simulink model "cruise_control_harness"  (Simulink 7.8)
settings: Solver=FixedStepDiscrete  SolverMode=SingleTasking  StartTime=0.0  StopTime=50  FixedStep=0.01  RelTol=1e-3  AbsTol=1e-6
model workspace (MAT data in the model file):
  converter_data = [0  137.465208994  2.232; 0.1  137.065019157  2.075; 0.2  135.864449646  1.975; 0.3  135.664354728  1.846; 0.4  137.565256453  1.72; 0.5  140.366585312  1.564; 0.6  145.268910814  1.409; 0.7  152.872517717  1.254; 0.8  162.9773111  1.096; 0.81  164.27792807  1.08; 0.82  166.178829795  1.061; 0.83  167.979684062  1.043; 0.84  170.080680706  1.028; 0.85  172.781962105  1.012; 0.86  175.383196045  1.002; 0.87  179.585189333  1.002; 0.88  183.587087703  1.001; 0.89  189.890077635  0.998; 0.9  197.693779455  0.999; 0.92  215.902417037  1.001; 0.94  244.515990379  1.002]
  emap = [-40  -44  -49  -53  -57  -61  -65  -70  -74  -78  -82; 215  117  85  66  44  29  10  -2  -13  -22  -32; 245  208  178  148  122  104  85  66  48  33  18; 264  260  241  219  193  167  152  133  119  96  85; 264  279  282  275  260  238  223  208  189  171  152; 267  290  293  297  290  275  260  256  234  212  193; 267  297  305  305  305  301  293  282  267  249  226; 267  301  308  312  319  323  319  316  297  279  253; 267  301  312  319  327  327  327  327  312  293  267; 267  301  312  319  327  334  334  334  319  305  275]
  Iei = 0.0219914882836
  nevec = [800 1200 1600 2000 2400 2800 3200 3600 4000 4400 4800]
  p0 = 0.07934
  p1 = 0.07934
  thvec = [0; 20; 30; 40; 50; 60; 70; 80; 90; 100]
  vehicledata : num (value not decoded)
values from neighbouring files (symbols this model uses):
  cruise_ki = 0.01    [cruise_control_data.m]    (also in fxpdata_simulinkpackage.mat)
  cruise_kp = 0.02    [cruise_control_data.m]    (also in fxpdata_simulinkpackage.mat)
  target_max = 100    [cruise_control_data.m]    (also in fxpdata_simulinkpackage.mat)
  target_min = 30    [cruise_control_data.m]    (also in fxpdata_simulinkpackage.mat)
  throt_max = 100    [cruise_control_data.m]    (also in fxpdata_simulinkpackage.mat)
  throt_min = 0    [cruise_control_data.m]    (also in fxpdata_simulinkpackage.mat)
  vel_dec = 1    [cruise_control_data.m]    (also in fxpdata_simulinkpackage.mat)
  vel_inc = 1    [cruise_control_data.m]    (also in fxpdata_simulinkpackage.mat)
undefined symbols (not defined in the file or in its folder): DiscIntNeverNeededParam, sigbuilder_block
libraries: simulink x2
settings Model: MinMaxOverflowLogging=MinMaxAndOverflow  SldvGeneratedHarnessModel=TestUnitModel=cruise_control|  Creator=The MathWorks Inc.  LastModifiedBy=itoy  RecordCoverage=on  CovSaveName=covdata_cc  CovMetricSettings=dcmtroe  CovHTMLOptions=-aTS=1 -bRG=1 -bTC=0 -hTR=0 -nFC=0 -scm=1 -bcm=1  CovModelRefEnable=off  CovExternalEMLEnable=on  ExtModeTrigMode=oneshot  ExtModeArmWhenConnect=off  ExtModeAutoUpdateStatusClock=off
settings DataIOCC: LimitDataPoints=off  SaveFormat=StructureWithTime  SaveOutput=off  SignalLogging=off  DSMLogging=off  SaveTime=off  SignalLoggingName=mysig
settings OptimizationCC: InlineParams=on  UseIntDivNetSlope=on  InlineInvariantSignals=on  EnhancedBackFolding=on  EfficientFloat2IntCast=on  OptimizeModelRefInitCode=on  LifeSpan=1
settings DebuggingCC: SignalInfNanChecking=error  SaveWithParameterizedLinksMsg=none  CheckExecutionContextPreStartOutputMsg=on  CheckExecutionContextRuntimeOutputMsg=on  SolverPrmCheckMsg=none  InheritedTsInSrcMsg=none  SingleTaskRateTransMsg=error  IntegerOverflowMsg=error  UniqueDataStoreMsg=error  BusObjectLabelMismatch=error  RootOutportRequireBusObject=error  AssertControl=DisableAll  StrictBusMsg=ErrorOnBusTreatedAsVector  BusNameAdapt=ErrorWithoutRepair  NonBusSignalsTreatedAsBus=error  LoggingUnavailableSignals=none
settings HardwareCC: ProdIntDivRoundTo=Zero  ProdEndianess=LittleEndian  ProdHWDeviceType=NEC->V850  TargetIntDivRoundTo=Zero  TargetEndianess=LittleEndian  TargetHWDeviceType=MATLAB Host
settings ModelReferenceCC: ModelReferenceNumInstancesAllowed=Single
settings SFSimCC: SFSimEcho=off  SimParseCustomCode=off
settings RTWCC: SystemTargetFile=ert.tlc  TemplateMakefile=ert_default_tmf  Description=Real-Time Workshop Embedded Coder  GenerateReport=on  ProcessScript=ert_make_rtw_hook  IncludeHyperlinkInReport=on  LaunchReport=on  IncludeERTFirstTime=on  RTWCompilerOptimization=On
settings CodeAppCC: IgnoreCustomStorageClasses=off
settings ERTTargetCC: MultiwordLength=2048  GenerateSampleERTMain=on  GenerateErtSFunction=on  CreateSILPILBlock=SIL  InlinedParameterPlacement=NonHierarchical  ERTCustomFileTemplate=example_file_process.tlc  ConvertIfToSwitch=off  SuppressUnreachableDefaultCases=off
settings ConfigComp: Description=Design Verifier Custom Configuration Component  DVMaxProcessTime=3000  DVDisplayUnsatisfiableObjectives=on  DVModelCoverageObjectives=MCDC  DVMaxTestCaseSteps=500  DVTestSuiteOptimization=CombinedObjectives  DVSaveReport=on

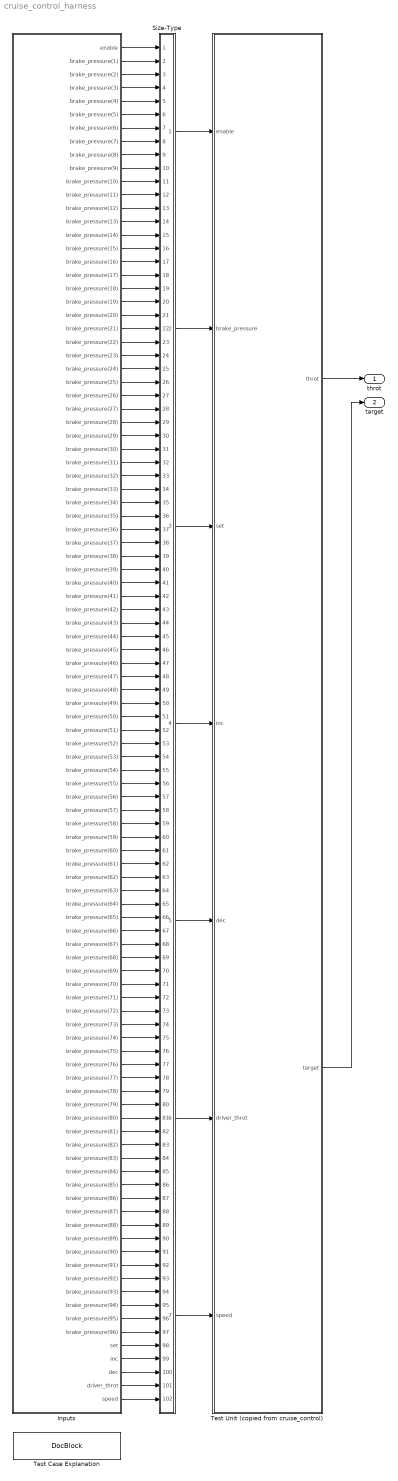
== system cruise_control_harness ==
  Inputs : Subsystem  Tag=STV Subsys  LoadFcn=sigbuilder_block('load',[49.5 50.25 519.75 399.75 ]);  StartFcn=sigbuilder_block('start');  StopFcn=sigbuilder_block('stop');  ClipboardFcn=sigbuilder_block('clipboard');  mask(Sigbuilder block){}
      mask init:
      | if ~strcmp(get_param(bdroot(gcb),'SimulationStatus'),'stopped'),tuvar = sigbuilder_block('maskInit'); end
      settings: CopyFcn=sigbuilder_block('copy');  DeleteFcn=sigbuilder_block('delete');  ModelCloseFcn=sigbuilder_block('modelClose');  PreSaveFcn=sigbuilder_block('preSave');  NameChangeFcn=sigbuilder_block('namechange');  OpenFcn=sigbuilder_block('open');  CloseFcn=sigbuilder_block('close');
      mask Display: plot(0, 0, 100, 100,[2, 2, 32, 32, 2], [68, 8, 8, 68, 68],[32, 2], [38, 38], [32, 19, 2],[53, 60, 44], [32, 17, 17, 2],[16, 16, 31, 31]);txt = getActiveGroup(gcbh);text(2, 100, txt,'verticalAlignment', 'top');
  Size-Type : Subsystem
  Test Case Explanation : simulink/Model-Wide Utilities/DocBlock  DocumentType=Text
  Test Unit (copied from cruise_control) : Subsystem
  throt : Outport  PortDimensions=[1 1]
  target : Outport  Port=2  PortDimensions=[1 1]
  wires:
  Inputs/1(enable) -> Size-Type/1(In1)
  Size-Type/1(Out1) -> Test Unit (copied from cruise_control)/1(enable)
  Inputs/2(brake_pressure(1)) -> Size-Type/2(In2)
  Inputs/3(brake_pressure(2)) -> Size-Type/3(In3)
  Inputs/4(brake_pressure(3)) -> Size-Type/4(In4)
  Inputs/5(brake_pressure(4)) -> Size-Type/5(In5)
  Inputs/6(brake_pressure(5)) -> Size-Type/6(In6)
  Inputs/7(brake_pressure(6)) -> Size-Type/7(In7)
  Inputs/8(brake_pressure(7)) -> Size-Type/8(In8)
  Inputs/9(brake_pressure(8)) -> Size-Type/9(In9)
  Inputs/10(brake_pressure(9)) -> Size-Type/10(In10)
  Inputs/11(brake_pressure(10)) -> Size-Type/11(In11)
  Inputs/12(brake_pressure(11)) -> Size-Type/12(In12)
  Inputs/13(brake_pressure(12)) -> Size-Type/13(In13)
  Inputs/14(brake_pressure(13)) -> Size-Type/14(In14)
  Inputs/15(brake_pressure(14)) -> Size-Type/15(In15)
  Inputs/16(brake_pressure(15)) -> Size-Type/16(In16)
  Inputs/17(brake_pressure(16)) -> Size-Type/17(In17)
  Inputs/18(brake_pressure(17)) -> Size-Type/18(In18)
  Inputs/19(brake_pressure(18)) -> Size-Type/19(In19)
  Inputs/20(brake_pressure(19)) -> Size-Type/20(In20)
  Inputs/21(brake_pressure(20)) -> Size-Type/21(In21)
  Inputs/22(brake_pressure(21)) -> Size-Type/22(In22)
  Inputs/23(brake_pressure(22)) -> Size-Type/23(In23)
  Inputs/24(brake_pressure(23)) -> Size-Type/24(In24)
  Inputs/25(brake_pressure(24)) -> Size-Type/25(In25)
  Inputs/26(brake_pressure(25)) -> Size-Type/26(In26)
  Inputs/27(brake_pressure(26)) -> Size-Type/27(In27)
  Inputs/28(brake_pressure(27)) -> Size-Type/28(In28)
  Inputs/29(brake_pressure(28)) -> Size-Type/29(In29)
  Inputs/30(brake_pressure(29)) -> Size-Type/30(In30)
  Inputs/31(brake_pressure(30)) -> Size-Type/31(In31)
  Inputs/32(brake_pressure(31)) -> Size-Type/32(In32)
  Inputs/33(brake_pressure(32)) -> Size-Type/33(In33)
  Inputs/34(brake_pressure(33)) -> Size-Type/34(In34)
  Inputs/35(brake_pressure(34)) -> Size-Type/35(In35)
  Inputs/36(brake_pressure(35)) -> Size-Type/36(In36)
  Inputs/37(brake_pressure(36)) -> Size-Type/37(In37)
  Inputs/38(brake_pressure(37)) -> Size-Type/38(In38)
  Inputs/39(brake_pressure(38)) -> Size-Type/39(In39)
  Inputs/40(brake_pressure(39)) -> Size-Type/40(In40)
  Inputs/41(brake_pressure(40)) -> Size-Type/41(In41)
  Inputs/42(brake_pressure(41)) -> Size-Type/42(In42)
  Inputs/43(brake_pressure(42)) -> Size-Type/43(In43)
  Inputs/44(brake_pressure(43)) -> Size-Type/44(In44)
  Inputs/45(brake_pressure(44)) -> Size-Type/45(In45)
  Inputs/46(brake_pressure(45)) -> Size-Type/46(In46)
  Inputs/47(brake_pressure(46)) -> Size-Type/47(In47)
  Inputs/48(brake_pressure(47)) -> Size-Type/48(In48)
  Inputs/49(brake_pressure(48)) -> Size-Type/49(In49)
  Inputs/50(brake_pressure(49)) -> Size-Type/50(In50)
  Inputs/51(brake_pressure(50)) -> Size-Type/51(In51)
  Inputs/52(brake_pressure(51)) -> Size-Type/52(In52)
  Inputs/53(brake_pressure(52)) -> Size-Type/53(In53)
  Inputs/54(brake_pressure(53)) -> Size-Type/54(In54)
  Inputs/55(brake_pressure(54)) -> Size-Type/55(In55)
  Inputs/56(brake_pressure(55)) -> Size-Type/56(In56)
  Inputs/57(brake_pressure(56)) -> Size-Type/57(In57)
  Inputs/58(brake_pressure(57)) -> Size-Type/58(In58)
  Inputs/59(brake_pressure(58)) -> Size-Type/59(In59)
  Inputs/60(brake_pressure(59)) -> Size-Type/60(In60)
  Inputs/61(brake_pressure(60)) -> Size-Type/61(In61)
  Inputs/62(brake_pressure(61)) -> Size-Type/62(In62)
  Inputs/63(brake_pressure(62)) -> Size-Type/63(In63)
  Inputs/64(brake_pressure(63)) -> Size-Type/64(In64)
  Inputs/65(brake_pressure(64)) -> Size-Type/65(In65)
  Inputs/66(brake_pressure(65)) -> Size-Type/66(In66)
  Inputs/67(brake_pressure(66)) -> Size-Type/67(In67)
  Inputs/68(brake_pressure(67)) -> Size-Type/68(In68)
  Inputs/69(brake_pressure(68)) -> Size-Type/69(In69)
  Inputs/70(brake_pressure(69)) -> Size-Type/70(In70)
  Inputs/71(brake_pressure(70)) -> Size-Type/71(In71)
  Inputs/72(brake_pressure(71)) -> Size-Type/72(In72)
  Inputs/73(brake_pressure(72)) -> Size-Type/73(In73)
  Inputs/74(brake_pressure(73)) -> Size-Type/74(In74)
  Inputs/75(brake_pressure(74)) -> Size-Type/75(In75)
  Inputs/76(brake_pressure(75)) -> Size-Type/76(In76)
  Inputs/77(brake_pressure(76)) -> Size-Type/77(In77)
  Inputs/78(brake_pressure(77)) -> Size-Type/78(In78)
  Inputs/79(brake_pressure(78)) -> Size-Type/79(In79)
  Inputs/80(brake_pressure(79)) -> Size-Type/80(In80)
  Inputs/81(brake_pressure(80)) -> Size-Type/81(In81)
  Inputs/82(brake_pressure(81)) -> Size-Type/82(In82)
  Inputs/83(brake_pressure(82)) -> Size-Type/83(In83)
  Inputs/84(brake_pressure(83)) -> Size-Type/84(In84)
  Inputs/85(brake_pressure(84)) -> Size-Type/85(In85)
  Inputs/86(brake_pressure(85)) -> Size-Type/86(In86)
  Inputs/87(brake_pressure(86)) -> Size-Type/87(In87)
  Inputs/88(brake_pressure(87)) -> Size-Type/88(In88)
  Inputs/89(brake_pressure(88)) -> Size-Type/89(In89)
  Inputs/90(brake_pressure(89)) -> Size-Type/90(In90)
  Inputs/91(brake_pressure(90)) -> Size-Type/91(In91)
  Inputs/92(brake_pressure(91)) -> Size-Type/92(In92)
  Inputs/93(brake_pressure(92)) -> Size-Type/93(In93)
  Inputs/94(brake_pressure(93)) -> Size-Type/94(In94)
  Inputs/95(brake_pressure(94)) -> Size-Type/95(In95)
  Inputs/96(brake_pressure(95)) -> Size-Type/96(In96)
  Inputs/97(brake_pressure(96)) -> Size-Type/97(In97)
  Size-Type/2(Out2) -> Test Unit (copied from cruise_control)/2(brake_pressure)
  Inputs/98(set) -> Size-Type/98(In98)
  Size-Type/3(Out3) -> Test Unit (copied from cruise_control)/3(set)
  Inputs/99(inc) -> Size-Type/99(In99)
  Size-Type/4(Out4) -> Test Unit (copied from cruise_control)/4(inc)
  Inputs/100(dec) -> Size-Type/100(In100)
  Size-Type/5(Out5) -> Test Unit (copied from cruise_control)/5(dec)
  Inputs/101(driver_throt) -> Size-Type/101(In101)
  Size-Type/6(Out6) -> Test Unit (copied from cruise_control)/6(driver_throt)
  Inputs/102(speed) -> Size-Type/102(In102)
  Size-Type/7(Out7) -> Test Unit (copied from cruise_control)/7(speed)
  Test Unit (copied from cruise_control)/1(throt) -> throt/1
  Test Unit (copied from cruise_control)/2(target) -> target/1

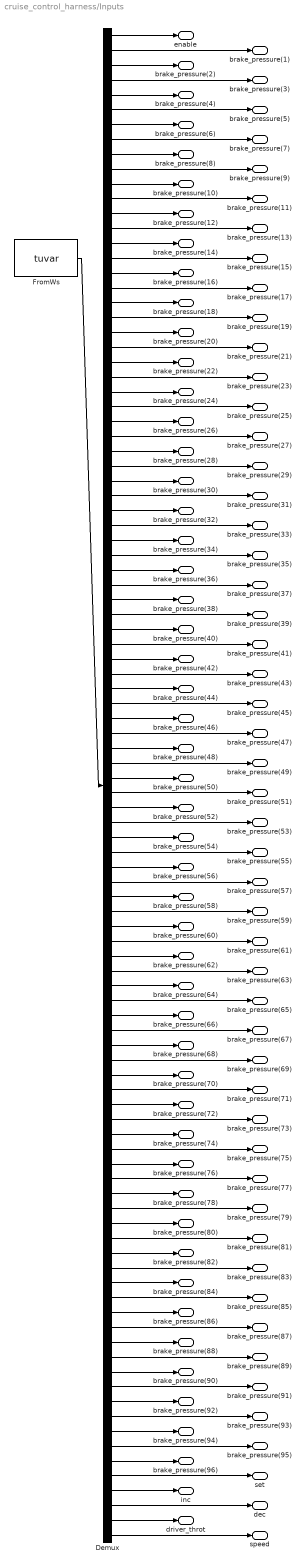
== system cruise_control_harness/Inputs ==
  Demux : Demux  Tag=STV Demux  Outputs=102
  FromWs : FromWorkspace  Tag=STV FromWs  VariableName=tuvar  SampleTime=0  SigBuilderData=DataTag1  VnvData=DataTag2
      SigBuilderData=|
      | dataSet.timeRange = [0 0.01]
      | dataSet.name = 'Test Case 1'
      | sbobj.Name = 'Signal Builder'
      | sbobj.Groups.Name = 'Test Case 1'
      | sbobj.Groups.Signals(1).Name = 'enable'
      | sbobj.Groups.Signals(1).XData = [0 0.01]
      | sbobj.Groups.Signals(1).YData = [0 0]
      | sbobj.Groups.Signals(2).Name = 'brake_pressure(1)'
      | sbobj.Groups.Signals(2).XData = [0 0.01]
      | sbobj.Groups.Signals(2).YData = [0 0]
      | sbobj.Groups.Signals(3).Name = 'brake_pressure(2)'
      | sbobj.Groups.Signals(3).XData = [0 0.01]
      | sbobj.Groups.Signals(3).YData = [0 0]
      | sbobj.Groups.Signals(4).Name = 'brake_pressure(3)'
      | sbobj.Groups.Signals(4).XData = [0 0.01]
      | sbobj.Groups.Signals(4).YData = [0 0]
      | sbobj.Groups.Signals(5).Name = 'brake_pressure(4)'
      | sbobj.Groups.Signals(5).XData = [0 0.01]
      | sbobj.Groups.Signals(5).YData = [0 0]
      | sbobj.Groups.Signals(6).Name = 'brake_pressure(5)'
      | sbobj.Groups.Signals(6).XData = [0 0.01]
      | sbobj.Groups.Signals(6).YData = [0 0]
      | sbobj.Groups.Signals(7).Name = 'brake_pressure(6)'
      | sbobj.Groups.Signals(7).XData = [0 0.01]
      | sbobj.Groups.Signals(7).YData = [0 0]
      | sbobj.Groups.Signals(8).Name = 'brake_pressure(7)'
      | sbobj.Groups.Signals(8).XData = [0 0.01]
      | sbobj.Groups.Signals(8).YData = [0 0]
      | sbobj.Groups.Signals(9).Name = 'brake_pressure(8)'
      | sbobj.Groups.Signals(9).XData = [0 0.01]
      | sbobj.Groups.Signals(9).YData = [0 0]
      | sbobj.Groups.Signals(10).Name = 'brake_pressure(9)'
      | sbobj.Groups.Signals(10).XData = [0 0.01]
      | sbobj.Groups.Signals(10).YData = [0 0]
      | sbobj.Groups.Signals(11).Name = 'brake_pressure(10)'
      | sbobj.Groups.Signals(11).XData = [0 0.01]
      | sbobj.Groups.Signals(11).YData = [0 0]
      | sbobj.Groups.Signals(12).Name = 'brake_pressure(11)'
      | sbobj.Groups.Signals(12).XData = [0 0.01]
      | sbobj.Groups.Signals(12).YData = [0 0]
      | sbobj.Groups.Signals(13).Name = 'brake_pressure(12)'
      | sbobj.Groups.Signals(13).XData = [0 0.01]
      | sbobj.Groups.Signals(13).YData = [0 0]
      | sbobj.Groups.Signals(14).Name = 'brake_pressure(13)'
      | sbobj.Groups.Signals(14).XData = [0 0.01]
      | sbobj.Groups.Signals(14).YData = [0 0]
      | sbobj.Groups.Signals(15).Name = 'brake_pressure(14)'
      | sbobj.Groups.Signals(15).XData = [0 0.01]
      | sbobj.Groups.Signals(15).YData = [0 0]
      | sbobj.Groups.Signals(16).Name = 'brake_pressure(15)'
      | sbobj.Groups.Signals(16).XData = [0 0.01]
      | sbobj.Groups.Signals(16).YData = [0 0]
      | sbobj.Groups.Signals(17).Name = 'brake_pressure(16)'
      | sbobj.Groups.Signals(17).XData = [0 0.01]
      | sbobj.Groups.Signals(17).YData = [0 0]
      | sbobj.Groups.Signals(18).Name = 'brake_pressure(17)'
      | sbobj.Groups.Signals(18).XData = [0 0.01]
      | sbobj.Groups.Signals(18).YData = [0 0]
      | sbobj.Groups.Signals(19).Name = 'brake_pressure(18)'
      | sbobj.Groups.Signals(19).XData = [0 0.01]
      | sbobj.Groups.Signals(19).YData = [0 0]
      | sbobj.Groups.Signals(20).Name = 'brake_pressure(19)'
      | sbobj.Groups.Signals(20).XData = [0 0.01]
      | sbobj.Groups.Signals(20).YData = [0 0]
      | sbobj.Groups.Signals(21).Name = 'brake_pressure(20)'
      | sbobj.Groups.Signals(21).XData = [0 0.01]
      | sbobj.Groups.Signals(21).YData = [0 0]
      | sbobj.Groups.Signals(22).Name = 'brake_pressure(21)'
      | sbobj.Groups.Signals(22).XData = [0 0.01]
      | sbobj.Groups.Signals(22).YData = [0 0]
      | sbobj.Groups.Signals(23).Name = 'brake_pressure(22)'
      | sbobj.Groups.Signals(23).XData = [0 0.01]
      | sbobj.Groups.Signals(23).YData = [0 0]
      | sbobj.Groups.Signals(24).Name = 'brake_pressure(23)'
      | sbobj.Groups.Signals(24).XData = [0 0.01]
      | sbobj.Groups.Signals(24).YData = [0 0]
      | sbobj.Groups.Signals(25).Name = 'brake_pressure(24)'
      | sbobj.Groups.Signals(25).XData = [0 0.01]
      | sbobj.Groups.Signals(25).YData = [0 0]
      | sbobj.Groups.Signals(26).Name = 'brake_pressure(25)'
      | sbobj.Groups.Signals(26).XData = [0 0.01]
      | sbobj.Groups.Signals(26).YData = [0 0]
      | sbobj.Groups.Signals(27).Name = 'brake_pressure(26)'
      | sbobj.Groups.Signals(27).XData = [0 0.01]
      | sbobj.Groups.Signals(27).YData = [0 0]
      | sbobj.Groups.Signals(28).Name = 'brake_pressure(27)'
      | sbobj.Groups.Signals(28).XData = [0 0.01]
      | sbobj.Groups.Signals(28).YData = [0 0]
      | sbobj.Groups.Signals(29).Name = 'brake_pressure(28)'
      | sbobj.Groups.Signals(29).XData = [0 0.01]
      | sbobj.Groups.Signals(29).YData = [0 0]
      | sbobj.Groups.Signals(30).Name = 'brake_pressure(29)'
      | sbobj.Groups.Signals(30).XData = [0 0.01]
      | sbobj.Groups.Signals(30).YData = [0 0]
      | sbobj.Groups.Signals(31).Name = 'brake_pressure(30)'
      | sbobj.Groups.Signals(31).XData = [0 0.01]
      | sbobj.Groups.Signals(31).YData = [0 0]
      | sbobj.Groups.Signals(32).Name = 'brake_pressure(31)'
      | sbobj.Groups.Signals(32).XData = [0 0.01]
      | sbobj.Groups.Signals(32).YData = [0 0]
      | sbobj.Groups.Signals(33).Name = 'brake_pressure(32)'
      | sbobj.Groups.Signals(33).XData = [0 0.01]
      | sbobj.Groups.Signals(33).YData = [0 0]
      | sbobj.Groups.Signals(34).Name = 'brake_pressure(33)'
      | sbobj.Groups.Signals(34).XData = [0 0.01]
      | sbobj.Groups.Signals(34).YData = [0 0]
      | sbobj.Groups.Signals(35).Name = 'brake_pressure(34)'
      | sbobj.Groups.Signals(35).XData = [0 0.01]
      | sbobj.Groups.Signals(35).YData = [0 0]
      | sbobj.Groups.Signals(36).Name = 'brake_pressure(35)'
      | sbobj.Groups.Signals(36).XData = [0 0.01]
      | sbobj.Groups.Signals(36).YData = [0 0]
      | sbobj.Groups.Signals(37).Name = 'brake_pressure(36)'
      | sbobj.Groups.Signals(37).XData = [0 0.01]
      | sbobj.Groups.Signals(37).YData = [0 0]
      | sbobj.Groups.Signals(38).Name = 'brake_pressure(37)'
      | sbobj.Groups.Signals(38).XData = [0 0.01]
      | sbobj.Groups.Signals(38).YData = [0 0]
      | sbobj.Groups.Signals(39).Name = 'brake_pressure(38)'
      | sbobj.Groups.Signals(39).XData = [0 0.01]
      | sbobj.Groups.Signals(39).YData = [0 0]
      | sbobj.Groups.Signals(40).Name = 'brake_pressure(39)'
      | sbobj.Groups.Signals(40).XData = [0 0.01]
      | sbobj.Groups.Signals(40).YData = [0 0]
      | sbobj.Groups.Signals(41).Name = 'brake_pressure(40)'
      | sbobj.Groups.Signals(41).XData = [0 0.01]
      | sbobj.Groups.Signals(41).YData = [0 0]
      | sbobj.Groups.Signals(42).Name = 'brake_pressure(41)'
      | sbobj.Groups.Signals(42).XData = [0 0.01]
      | sbobj.Groups.Signals(42).YData = [0 0]
      | sbobj.Groups.Signals(43).Name = 'brake_pressure(42)'
      | sbobj.Groups.Signals(43).XData = [0 0.01]
      | sbobj.Groups.Signals(43).YData = [0 0]
      | sbobj.Groups.Signals(44).Name = 'brake_pressure(43)'
      | sbobj.Groups.Signals(44).XData = [0 0.01]
      | sbobj.Groups.Signals(44).YData = [0 0]
      | sbobj.Groups.Signals(45).Name = 'brake_pressure(44)'
      | sbobj.Groups.Signals(45).XData = [0 0.01]
      | sbobj.Groups.Signals(45).YData = [0 0]
      | sbobj.Groups.Signals(46).Name = 'brake_pressure(45)'
      | sbobj.Groups.Signals(46).XData = [0 0.01]
      | sbobj.Groups.Signals(46).YData = [0 0]
      | sbobj.Groups.Signals(47).Name = 'brake_pressure(46)'
      | sbobj.Groups.Signals(47).XData = [0 0.01]
      | sbobj.Groups.Signals(47).YData = [0 0]
      | sbobj.Groups.Signals(48).Name = 'brake_pressure(47)'
      | sbobj.Groups.Signals(48).XData = [0 0.01]
      | sbobj.Groups.Signals(48).YData = [0 0]
      | sbobj.Groups.Signals(49).Name = 'brake_pressure(48)'
      | sbobj.Groups.Signals(49).XData = [0 0.01]
      | sbobj.Groups.Signals(49).YData = [0 0]
      | sbobj.Groups.Signals(50).Name = 'brake_pressure(49)'
      | sbobj.Groups.Signals(50).XData = [0 0.01]
      | sbobj.Groups.Signals(50).YData = [0 0]
      | sbobj.Groups.Signals(51).Name = 'brake_pressure(50)'
      | sbobj.Groups.Signals(51).XData = [0 0.01]
      | sbobj.Groups.Signals(51).YData = [0 0]
      | sbobj.Groups.Signals(52).Name = 'brake_pressure(51)'
      | sbobj.Groups.Signals(52).XData = [0 0.01]
      | sbobj.Groups.Signals(52).YData = [0 0]
      | sbobj.Groups.Signals(53).Name = 'brake_pressure(52)'
      | sbobj.Groups.Signals(53).XData = [0 0.01]
      | sbobj.Groups.Signals(53).YData = [0 0]
      | sbobj.Groups.Signals(54).Name = 'brake_pressure(53)'
      | sbobj.Groups.Signals(54).XData = [0 0.01]
      | sbobj.Groups.Signals(54).YData = [0 0]
      | sbobj.Groups.Signals(55).Name = 'brake_pressure(54)'
      | sbobj.Groups.Signals(55).XData = [0 0.01]
      | sbobj.Groups.Signals(55).YData = [0 0]
      | sbobj.Groups.Signals(56).Name = 'brake_pressure(55)'
      | sbobj.Groups.Signals(56).XData = [0 0.01]
      | sbobj.Groups.Signals(56).YData = [0 0]
      | sbobj.Groups.Signals(57).Name = 'brake_pressure(56)'
      | sbobj.Groups.Signals(57).XData = [0 0.01]
      | sbobj.Groups.Signals(57).YData = [0 0]
      | sbobj.Groups.Signals(58).Name = 'brake_pressure(57)'
      | sbobj.Groups.Signals(58).XData = [0 0.01]
      | sbobj.Groups.Signals(58).YData = [0 0]
      | sbobj.Groups.Signals(59).Name = 'brake_pressure(58)'
      | sbobj.Groups.Signals(59).XData = [0 0.01]
      | sbobj.Groups.Signals(59).YData = [0 0]
      | sbobj.Groups.Signals(60).Name = 'brake_pressure(59)'
      | sbobj.Groups.Signals(60).XData = [0 0.01]
      | sbobj.Groups.Signals(60).YData = [0 0]
      | sbobj.Groups.Signals(61).Name = 'brake_pressure(60)'
      | sbobj.Groups.Signals(61).XData = [0 0.01]
      | sbobj.Groups.Signals(61).YData = [0 0]
      | sbobj.Groups.Signals(62).Name = 'brake_pressure(61)'
      | sbobj.Groups.Signals(62).XData = [0 0.01]
      | sbobj.Groups.Signals(62).YData = [0 0]
      | sbobj.Groups.Signals(63).Name = 'brake_pressure(62)'
      | sbobj.Groups.Signals(63).XData = [0 0.01]
      | sbobj.Groups.Signals(63).YData = [0 0]
      | sbobj.Groups.Signals(64).Name = 'brake_pressure(63)'
      | sbobj.Groups.Signals(64).XData = [0 0.01]
      | sbobj.Groups.Signals(64).YData = [0 0]
      | sbobj.Groups.Signals(65).Name = 'brake_pressure(64)'
      | sbobj.Groups.Signals(65).XData = [0 0.01]
      | sbobj.Groups.Signals(65).YData = [0 0]
      | sbobj.Groups.Signals(66).Name = 'brake_pressure(65)'
      | sbobj.Groups.Signals(66).XData = [0 0.01]
      | sbobj.Groups.Signals(66).YData = [0 0]
      | sbobj.Groups.Signals(67).Name = 'brake_pressure(66)'
      | sbobj.Groups.Signals(67).XData = [0 0.01]
      | sbobj.Groups.Signals(67).YData = [0 0]
      | sbobj.Groups.Signals(68).Name = 'brake_pressure(67)'
      | sbobj.Groups.Signals(68).XData = [0 0.01]
      | sbobj.Groups.Signals(68).YData = [0 0]
      | sbobj.Groups.Signals(69).Name = 'brake_pressure(68)'
      | sbobj.Groups.Signals(69).XData = [0 0.01]
      | sbobj.Groups.Signals(69).YData = [0 0]
      | sbobj.Groups.Signals(70).Name = 'brake_pressure(69)'
      | sbobj.Groups.Signals(70).XData = [0 0.01]
      | sbobj.Groups.Signals(70).YData = [0 0]
      | sbobj.Groups.Signals(71).Name = 'brake_pressure(70)'
      | sbobj.Groups.Signals(71).XData = [0 0.01]
      | sbobj.Groups.Signals(71).YData = [0 0]
      | sbobj.Groups.Signals(72).Name = 'brake_pressure(71)'
      | sbobj.Groups.Signals(72).XData = [0 0.01]
      | sbobj.Groups.Signals(72).YData = [0 0]
      | sbobj.Groups.Signals(73).Name = 'brake_pressure(72)'
      | sbobj.Groups.Signals(73).XData = [0 0.01]
      | sbobj.Groups.Signals(73).YData = [0 0]
      | sbobj.Groups.Signals(74).Name = 'brake_pressure(73)'
      | sbobj.Groups.Signals(74).XData = [0 0.01]
      | sbobj.Groups.Signals(74).YData = [0 0]
      | sbobj.Groups.Signals(75).Name = 'brake_pressure(74)'
      | sbobj.Groups.Signals(75).XData = [0 0.01]
      | sbobj.Groups.Signals(75).YData = [0 0]
      | sbobj.Groups.Signals(76).Name = 'brake_pressure(75)'
      | sbobj.Groups.Signals(76).XData = [0 0.01]
      | sbobj.Groups.Signals(76).YData = [0 0]
      | sbobj.Groups.Signals(77).Name = 'brake_pressure(76)'
      | sbobj.Groups.Signals(77).XData = [0 0.01]
      | sbobj.Groups.Signals(77).YData = [0 0]
      | sbobj.Groups.Signals(78).Name = 'brake_pressure(77)'
      | sbobj.Groups.Signals(78).XData = [0 0.01]
      | sbobj.Groups.Signals(78).YData = [0 0]
      | sbobj.Groups.Signals(79).Name = 'brake_pressure(78)'
      | sbobj.Groups.Signals(79).XData = [0 0.01]
      | sbobj.Groups.Signals(79).YData = [0 0]
      | sbobj.Groups.Signals(80).Name = 'brake_pressure(79)'
      | sbobj.Groups.Signals(80).XData = [0 0.01]
      | sbobj.Groups.Signals(80).YData = [0 0]
      | sbobj.Groups.Signals(81).Name = 'brake_pressure(80)'
      | sbobj.Groups.Signals(81).XData = [0 0.01]
      | sbobj.Groups.Signals(81).YData = [0 0]
      | sbobj.Groups.Signals(82).Name = 'brake_pressure(81)'
      | sbobj.Groups.Signals(82).XData = [0 0.01]
      | sbobj.Groups.Signals(82).YData = [0 0]
      | sbobj.Groups.Signals(83).Name = 'brake_pressure(82)'
      | sbobj.Groups.Signals(83).XData = [0 0.01]
      | sbobj.Groups.Signals(83).YData = [0 0]
      | sbobj.Groups.Signals(84).Name = 'brake_pressure(83)'
      | sbobj.Groups.Signals(84).XData = [0 0.01]
      | sbobj.Groups.Signals(84).YData = [0 0]
      | sbobj.Groups.Signals(85).Name = 'brake_pressure(84)'
      | sbobj.Groups.Signals(85).XData = [0 0.01]
      | sbobj.Groups.Signals(85).YData = [0 0]
      | sbobj.Groups.Signals(86).Name = 'brake_pressure(85)'
      | sbobj.Groups.Signals(86).XData = [0 0.01]
      | sbobj.Groups.Signals(86).YData = [0 0]
      | sbobj.Groups.Signals(87).Name = 'brake_pressure(86)'
      | sbobj.Groups.Signals(87).XData = [0 0.01]
      | sbobj.Groups.Signals(87).YData = [0 0]
      | sbobj.Groups.Signals(88).Name = 'brake_pressure(87)'
      | sbobj.Groups.Signals(88).XData = [0 0.01]
      | sbobj.Groups.Signals(88).YData = [0 0]
      | sbobj.Groups.Signals(89).Name = 'brake_pressure(88)'
      | sbobj.Groups.Signals(89).XData = [0 0.01]
      | sbobj.Groups.Signals(89).YData = [0 0]
      | sbobj.Groups.Signals(90).Name = 'brake_pressure(89)'
      | sbobj.Groups.Signals(90).XData = [0 0.01]
      | sbobj.Groups.Signals(90).YData = [0 0]
      | sbobj.Groups.Signals(91).Name = 'brake_pressure(90)'
      | sbobj.Groups.Signals(91).XData = [0 0.01]
      | sbobj.Groups.Signals(91).YData = [0 0]
      | sbobj.Groups.Signals(92).Name = 'brake_pressure(91)'
      | sbobj.Groups.Signals(92).XData = [0 0.01]
      | sbobj.Groups.Signals(92).YData = [0 0]
      | sbobj.Groups.Signals(93).Name = 'brake_pressure(92)'
      | sbobj.Groups.Signals(93).XData = [0 0.01]
      | sbobj.Groups.Signals(93).YData = [0 0]
      | sbobj.Groups.Signals(94).Name = 'brake_pressure(93)'
      | sbobj.Groups.Signals(94).XData = [0 0.01]
      | sbobj.Groups.Signals(94).YData = [0 0]
      | sbobj.Groups.Signals(95).Name = 'brake_pressure(94)'
      | sbobj.Groups.Signals(95).XData = [0 0.01]
      | sbobj.Groups.Signals(95).YData = [0 0]
      | sbobj.Groups.Signals(96).Name = 'brake_pressure(95)'
      | sbobj.Groups.Signals(96).XData = [0 0.01]
      | sbobj.Groups.Signals(96).YData = [0 0]
      | sbobj.Groups.Signals(97).Name = 'brake_pressure(96)'
      | sbobj.Groups.Signals(97).XData = [0 0.01]
      | sbobj.Groups.Signals(97).YData = [0 0]
      | sbobj.Groups.Signals(98).Name = 'set'
      | sbobj.Groups.Signals(98).XData = [0 0.01]
      | sbobj.Groups.Signals(98).YData = [0 0]
      | sbobj.Groups.Signals(99).Name = 'inc'
      | sbobj.Groups.Signals(99).XData = [0 0.01]
      | sbobj.Groups.Signals(99).YData = [0 0]
      | sbobj.Groups.Signals(100).Name = 'dec'
      | sbobj.Groups.Signals(100).XData = [0 0.01]
      | sbobj.Groups.Signals(100).YData = [0 0]
      | sbobj.Groups.Signals(101).Name = 'driver_throt'
      | sbobj.Groups.Signals(101).XData = [0 0.01]
      | sbobj.Groups.Signals(101).YData = [0 0]
      | sbobj.Groups.Signals(102).Name = 'speed'
      | sbobj.Groups.Signals(102).XData = [0 0.01]
      | sbobj.Groups.Signals(102).YData = [0 0]
      | sbobj.Groups.TimeRange = [0 0.01]
  enable : Outport  Tag=STV Outport
  brake_pressure(1) : Outport  Tag=STV Outport  Port=2
  brake_pressure(2) : Outport  Tag=STV Outport  Port=3
  brake_pressure(3) : Outport  Tag=STV Outport  Port=4
  brake_pressure(4) : Outport  Tag=STV Outport  Port=5
  brake_pressure(5) : Outport  Tag=STV Outport  Port=6
  brake_pressure(6) : Outport  Tag=STV Outport  Port=7
  brake_pressure(7) : Outport  Tag=STV Outport  Port=8
  brake_pressure(8) : Outport  Tag=STV Outport  Port=9
  brake_pressure(9) : Outport  Tag=STV Outport  Port=10
  brake_pressure(10) : Outport  Tag=STV Outport  Port=11
  brake_pressure(11) : Outport  Tag=STV Outport  Port=12
  brake_pressure(12) : Outport  Tag=STV Outport  Port=13
  brake_pressure(13) : Outport  Tag=STV Outport  Port=14
  brake_pressure(14) : Outport  Tag=STV Outport  Port=15
  brake_pressure(15) : Outport  Tag=STV Outport  Port=16
  brake_pressure(16) : Outport  Tag=STV Outport  Port=17
  brake_pressure(17) : Outport  Tag=STV Outport  Port=18
  brake_pressure(18) : Outport  Tag=STV Outport  Port=19
  brake_pressure(19) : Outport  Tag=STV Outport  Port=20
  brake_pressure(20) : Outport  Tag=STV Outport  Port=21
  brake_pressure(21) : Outport  Tag=STV Outport  Port=22
  brake_pressure(22) : Outport  Tag=STV Outport  Port=23
  brake_pressure(23) : Outport  Tag=STV Outport  Port=24
  brake_pressure(24) : Outport  Tag=STV Outport  Port=25
  brake_pressure(25) : Outport  Tag=STV Outport  Port=26
  brake_pressure(26) : Outport  Tag=STV Outport  Port=27
  brake_pressure(27) : Outport  Tag=STV Outport  Port=28
  brake_pressure(28) : Outport  Tag=STV Outport  Port=29
  brake_pressure(29) : Outport  Tag=STV Outport  Port=30
  brake_pressure(30) : Outport  Tag=STV Outport  Port=31
  brake_pressure(31) : Outport  Tag=STV Outport  Port=32
  brake_pressure(32) : Outport  Tag=STV Outport  Port=33
  brake_pressure(33) : Outport  Tag=STV Outport  Port=34
  brake_pressure(34) : Outport  Tag=STV Outport  Port=35
  brake_pressure(35) : Outport  Tag=STV Outport  Port=36
  brake_pressure(36) : Outport  Tag=STV Outport  Port=37
  brake_pressure(37) : Outport  Tag=STV Outport  Port=38
  brake_pressure(38) : Outport  Tag=STV Outport  Port=39
  brake_pressure(39) : Outport  Tag=STV Outport  Port=40
  brake_pressure(40) : Outport  Tag=STV Outport  Port=41
  brake_pressure(41) : Outport  Tag=STV Outport  Port=42
  brake_pressure(42) : Outport  Tag=STV Outport  Port=43
  brake_pressure(43) : Outport  Tag=STV Outport  Port=44
  brake_pressure(44) : Outport  Tag=STV Outport  Port=45
  brake_pressure(45) : Outport  Tag=STV Outport  Port=46
  brake_pressure(46) : Outport  Tag=STV Outport  Port=47
  brake_pressure(47) : Outport  Tag=STV Outport  Port=48
  brake_pressure(48) : Outport  Tag=STV Outport  Port=49
  brake_pressure(49) : Outport  Tag=STV Outport  Port=50
  brake_pressure(50) : Outport  Tag=STV Outport  Port=51
  brake_pressure(51) : Outport  Tag=STV Outport  Port=52
  brake_pressure(52) : Outport  Tag=STV Outport  Port=53
  brake_pressure(53) : Outport  Tag=STV Outport  Port=54
  brake_pressure(54) : Outport  Tag=STV Outport  Port=55
  brake_pressure(55) : Outport  Tag=STV Outport  Port=56
  brake_pressure(56) : Outport  Tag=STV Outport  Port=57
  brake_pressure(57) : Outport  Tag=STV Outport  Port=58
  brake_pressure(58) : Outport  Tag=STV Outport  Port=59
  brake_pressure(59) : Outport  Tag=STV Outport  Port=60
  brake_pressure(60) : Outport  Tag=STV Outport  Port=61
  brake_pressure(61) : Outport  Tag=STV Outport  Port=62
  brake_pressure(62) : Outport  Tag=STV Outport  Port=63
  brake_pressure(63) : Outport  Tag=STV Outport  Port=64
  brake_pressure(64) : Outport  Tag=STV Outport  Port=65
  brake_pressure(65) : Outport  Tag=STV Outport  Port=66
  brake_pressure(66) : Outport  Tag=STV Outport  Port=67
  brake_pressure(67) : Outport  Tag=STV Outport  Port=68
  brake_pressure(68) : Outport  Tag=STV Outport  Port=69
  brake_pressure(69) : Outport  Tag=STV Outport  Port=70
  brake_pressure(70) : Outport  Tag=STV Outport  Port=71
  brake_pressure(71) : Outport  Tag=STV Outport  Port=72
  brake_pressure(72) : Outport  Tag=STV Outport  Port=73
  brake_pressure(73) : Outport  Tag=STV Outport  Port=74
  brake_pressure(74) : Outport  Tag=STV Outport  Port=75
  brake_pressure(75) : Outport  Tag=STV Outport  Port=76
  brake_pressure(76) : Outport  Tag=STV Outport  Port=77
  brake_pressure(77) : Outport  Tag=STV Outport  Port=78
  brake_pressure(78) : Outport  Tag=STV Outport  Port=79
  brake_pressure(79) : Outport  Tag=STV Outport  Port=80
  brake_pressure(80) : Outport  Tag=STV Outport  Port=81
  brake_pressure(81) : Outport  Tag=STV Outport  Port=82
  brake_pressure(82) : Outport  Tag=STV Outport  Port=83
  brake_pressure(83) : Outport  Tag=STV Outport  Port=84
  brake_pressure(84) : Outport  Tag=STV Outport  Port=85
  brake_pressure(85) : Outport  Tag=STV Outport  Port=86
  brake_pressure(86) : Outport  Tag=STV Outport  Port=87
  brake_pressure(87) : Outport  Tag=STV Outport  Port=88
  brake_pressure(88) : Outport  Tag=STV Outport  Port=89
  brake_pressure(89) : Outport  Tag=STV Outport  Port=90
  brake_pressure(90) : Outport  Tag=STV Outport  Port=91
  brake_pressure(91) : Outport  Tag=STV Outport  Port=92
  brake_pressure(92) : Outport  Tag=STV Outport  Port=93
  brake_pressure(93) : Outport  Tag=STV Outport  Port=94
  brake_pressure(94) : Outport  Tag=STV Outport  Port=95
  brake_pressure(95) : Outport  Tag=STV Outport  Port=96
  brake_pressure(96) : Outport  Tag=STV Outport  Port=97
  set : Outport  Tag=STV Outport  Port=98
  inc : Outport  Tag=STV Outport  Port=99
  dec : Outport  Tag=STV Outport  Port=100
  driver_throt : Outport  Tag=STV Outport  Port=101
  speed : Outport  Tag=STV Outport  Port=102
  wires:
  FromWs/1 -> Demux/1
  Demux/1 -> enable/1
  Demux/2 -> brake_pressure(1)/1
  Demux/3 -> brake_pressure(2)/1
  Demux/4 -> brake_pressure(3)/1
  Demux/5 -> brake_pressure(4)/1
  Demux/6 -> brake_pressure(5)/1
  Demux/7 -> brake_pressure(6)/1
  Demux/8 -> brake_pressure(7)/1
  Demux/9 -> brake_pressure(8)/1
  Demux/10 -> brake_pressure(9)/1
  Demux/11 -> brake_pressure(10)/1
  Demux/12 -> brake_pressure(11)/1
  Demux/13 -> brake_pressure(12)/1
  Demux/14 -> brake_pressure(13)/1
  Demux/15 -> brake_pressure(14)/1
  Demux/16 -> brake_pressure(15)/1
  Demux/17 -> brake_pressure(16)/1
  Demux/18 -> brake_pressure(17)/1
  Demux/19 -> brake_pressure(18)/1
  Demux/20 -> brake_pressure(19)/1
  Demux/21 -> brake_pressure(20)/1
  Demux/22 -> brake_pressure(21)/1
  Demux/23 -> brake_pressure(22)/1
  Demux/24 -> brake_pressure(23)/1
  Demux/25 -> brake_pressure(24)/1
  Demux/26 -> brake_pressure(25)/1
  Demux/27 -> brake_pressure(26)/1
  Demux/28 -> brake_pressure(27)/1
  Demux/29 -> brake_pressure(28)/1
  Demux/30 -> brake_pressure(29)/1
  Demux/31 -> brake_pressure(30)/1
  Demux/32 -> brake_pressure(31)/1
  Demux/33 -> brake_pressure(32)/1
  Demux/34 -> brake_pressure(33)/1
  Demux/35 -> brake_pressure(34)/1
  Demux/36 -> brake_pressure(35)/1
  Demux/37 -> brake_pressure(36)/1
  Demux/38 -> brake_pressure(37)/1
  Demux/39 -> brake_pressure(38)/1
  Demux/40 -> brake_pressure(39)/1
  Demux/41 -> brake_pressure(40)/1
  Demux/42 -> brake_pressure(41)/1
  Demux/43 -> brake_pressure(42)/1
  Demux/44 -> brake_pressure(43)/1
  Demux/45 -> brake_pressure(44)/1
  Demux/46 -> brake_pressure(45)/1
  Demux/47 -> brake_pressure(46)/1
  Demux/48 -> brake_pressure(47)/1
  Demux/49 -> brake_pressure(48)/1
  Demux/50 -> brake_pressure(49)/1
  Demux/51 -> brake_pressure(50)/1
  Demux/52 -> brake_pressure(51)/1
  Demux/53 -> brake_pressure(52)/1
  Demux/54 -> brake_pressure(53)/1
  Demux/55 -> brake_pressure(54)/1
  Demux/56 -> brake_pressure(55)/1
  Demux/57 -> brake_pressure(56)/1
  Demux/58 -> brake_pressure(57)/1
  Demux/59 -> brake_pressure(58)/1
  Demux/60 -> brake_pressure(59)/1
  Demux/61 -> brake_pressure(60)/1
  Demux/62 -> brake_pressure(61)/1
  Demux/63 -> brake_pressure(62)/1
  Demux/64 -> brake_pressure(63)/1
  Demux/65 -> brake_pressure(64)/1
  Demux/66 -> brake_pressure(65)/1
  Demux/67 -> brake_pressure(66)/1
  Demux/68 -> brake_pressure(67)/1
  Demux/69 -> brake_pressure(68)/1
  Demux/70 -> brake_pressure(69)/1
  Demux/71 -> brake_pressure(70)/1
  Demux/72 -> brake_pressure(71)/1
  Demux/73 -> brake_pressure(72)/1
  Demux/74 -> brake_pressure(73)/1
  Demux/75 -> brake_pressure(74)/1
  Demux/76 -> brake_pressure(75)/1
  Demux/77 -> brake_pressure(76)/1
  Demux/78 -> brake_pressure(77)/1
  Demux/79 -> brake_pressure(78)/1
  Demux/80 -> brake_pressure(79)/1
  Demux/81 -> brake_pressure(80)/1
  Demux/82 -> brake_pressure(81)/1
  Demux/83 -> brake_pressure(82)/1
  Demux/84 -> brake_pressure(83)/1
  Demux/85 -> brake_pressure(84)/1
  Demux/86 -> brake_pressure(85)/1
  Demux/87 -> brake_pressure(86)/1
  Demux/88 -> brake_pressure(87)/1
  Demux/89 -> brake_pressure(88)/1
  Demux/90 -> brake_pressure(89)/1
  Demux/91 -> brake_pressure(90)/1
  Demux/92 -> brake_pressure(91)/1
  Demux/93 -> brake_pressure(92)/1
  Demux/94 -> brake_pressure(93)/1
  Demux/95 -> brake_pressure(94)/1
  Demux/96 -> brake_pressure(95)/1
  Demux/97 -> brake_pressure(96)/1
  Demux/98 -> set/1
  Demux/99 -> inc/1
  Demux/100 -> dec/1
  Demux/101 -> driver_throt/1
  Demux/102 -> speed/1

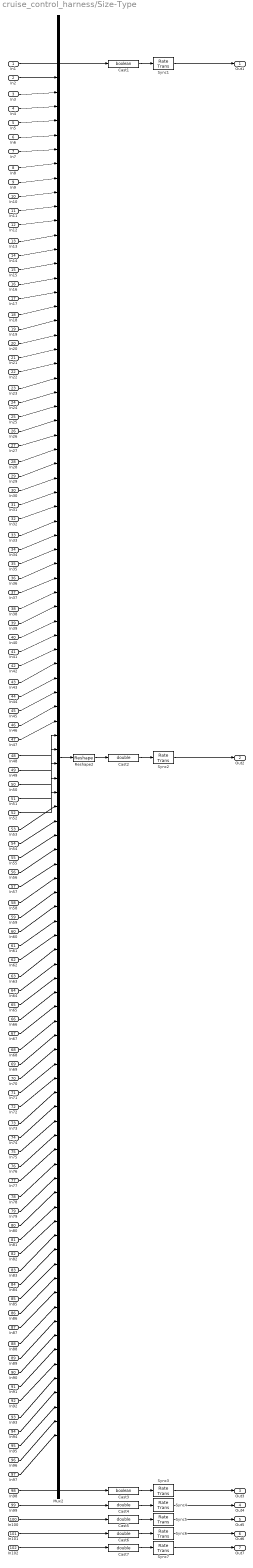
== system cruise_control_harness/Size-Type ==
  In1 : Inport
  In2 : Inport  Port=2
  In3 : Inport  Port=3
  In4 : Inport  Port=4
  In5 : Inport  Port=5
  In6 : Inport  Port=6
  In7 : Inport  Port=7
  In8 : Inport  Port=8
  In9 : Inport  Port=9
  In10 : Inport  Port=10
  In11 : Inport  Port=11
  In12 : Inport  Port=12
  In13 : Inport  Port=13
  In14 : Inport  Port=14
  In15 : Inport  Port=15
  In16 : Inport  Port=16
  In17 : Inport  Port=17
  In18 : Inport  Port=18
  In19 : Inport  Port=19
  In20 : Inport  Port=20
  In21 : Inport  Port=21
  In22 : Inport  Port=22
  In23 : Inport  Port=23
  In24 : Inport  Port=24
  In25 : Inport  Port=25
  In26 : Inport  Port=26
  In27 : Inport  Port=27
  In28 : Inport  Port=28
  In29 : Inport  Port=29
  In30 : Inport  Port=30
  In31 : Inport  Port=31
  In32 : Inport  Port=32
  In33 : Inport  Port=33
  In34 : Inport  Port=34
  In35 : Inport  Port=35
  In36 : Inport  Port=36
  In37 : Inport  Port=37
  In38 : Inport  Port=38
  In39 : Inport  Port=39
  In40 : Inport  Port=40
  In41 : Inport  Port=41
  In42 : Inport  Port=42
  In43 : Inport  Port=43
  In44 : Inport  Port=44
  In45 : Inport  Port=45
  In46 : Inport  Port=46
  In47 : Inport  Port=47
  In48 : Inport  Port=48
  In49 : Inport  Port=49
  In50 : Inport  Port=50
  In51 : Inport  Port=51
  In52 : Inport  Port=52
  In53 : Inport  Port=53
  In54 : Inport  Port=54
  In55 : Inport  Port=55
  In56 : Inport  Port=56
  In57 : Inport  Port=57
  In58 : Inport  Port=58
  In59 : Inport  Port=59
  In60 : Inport  Port=60
  In61 : Inport  Port=61
  In62 : Inport  Port=62
  In63 : Inport  Port=63
  In64 : Inport  Port=64
  In65 : Inport  Port=65
  In66 : Inport  Port=66
  In67 : Inport  Port=67
  In68 : Inport  Port=68
  In69 : Inport  Port=69
  In70 : Inport  Port=70
  In71 : Inport  Port=71
  In72 : Inport  Port=72
  In73 : Inport  Port=73
  In74 : Inport  Port=74
  In75 : Inport  Port=75
  In76 : Inport  Port=76
  In77 : Inport  Port=77
  In78 : Inport  Port=78
  In79 : Inport  Port=79
  In80 : Inport  Port=80
  In81 : Inport  Port=81
  In82 : Inport  Port=82
  In83 : Inport  Port=83
  In84 : Inport  Port=84
  In85 : Inport  Port=85
  In86 : Inport  Port=86
  In87 : Inport  Port=87
  In88 : Inport  Port=88
  In89 : Inport  Port=89
  In90 : Inport  Port=90
  In91 : Inport  Port=91
  In92 : Inport  Port=92
  In93 : Inport  Port=93
  In94 : Inport  Port=94
  In95 : Inport  Port=95
  In96 : Inport  Port=96
  In97 : Inport  Port=97
  In98 : Inport  Port=98
  In99 : Inport  Port=99
  In100 : Inport  Port=100
  In101 : Inport  Port=101
  In102 : Inport  Port=102
  Cast1 : DataTypeConversion  OutDataTypeStr=boolean  SaturateOnIntegerOverflow=on  RndMeth=Zero
  Cast{2,4..7} (5 alike) : DataTypeConversion  OutDataTypeStr=double  SaturateOnIntegerOverflow=on  RndMeth=Zero
  Cast3 : DataTypeConversion  OutDataTypeStr=boolean  SaturateOnIntegerOverflow=on  RndMeth=Zero
  Mux2 : Mux  Inputs=96
  Reshape2 : Reshape  OutputDimensionality=Customize  OutputDimensions=96
  Sync{1..7} (7 alike) : RateTransition  OutPortSampleTime=[0.01,0]
  Out1 : Outport
  Out2 : Outport  Port=2
  Out3 : Outport  Port=3
  Out4 : Outport  Port=4
  Out5 : Outport  Port=5
  Out6 : Outport  Port=6
  Out7 : Outport  Port=7
  wires:
  In1/1 -> Cast1/1
  Cast1/1 -> Sync1/1
  Sync1/1 -> Out1/1
  In2/1 -> Mux2/1
  In3/1 -> Mux2/2
  In4/1 -> Mux2/3
  In5/1 -> Mux2/4
  In6/1 -> Mux2/5
  In7/1 -> Mux2/6
  In8/1 -> Mux2/7
  In9/1 -> Mux2/8
  In10/1 -> Mux2/9
  In11/1 -> Mux2/10
  In12/1 -> Mux2/11
  In13/1 -> Mux2/12
  In14/1 -> Mux2/13
  In15/1 -> Mux2/14
  In16/1 -> Mux2/15
  In17/1 -> Mux2/16
  In18/1 -> Mux2/17
  In19/1 -> Mux2/18
  In20/1 -> Mux2/19
  In21/1 -> Mux2/20
  In22/1 -> Mux2/21
  In23/1 -> Mux2/22
  In24/1 -> Mux2/23
  In25/1 -> Mux2/24
  In26/1 -> Mux2/25
  In27/1 -> Mux2/26
  In28/1 -> Mux2/27
  In29/1 -> Mux2/28
  In30/1 -> Mux2/29
  In31/1 -> Mux2/30
  In32/1 -> Mux2/31
  In33/1 -> Mux2/32
  In34/1 -> Mux2/33
  In35/1 -> Mux2/34
  In36/1 -> Mux2/35
  In37/1 -> Mux2/36
  In38/1 -> Mux2/37
  In39/1 -> Mux2/38
  In40/1 -> Mux2/39
  In41/1 -> Mux2/40
  In42/1 -> Mux2/41
  In43/1 -> Mux2/42
  In44/1 -> Mux2/43
  In45/1 -> Mux2/44
  In46/1 -> Mux2/45
  In47/1 -> Mux2/46
  In48/1 -> Mux2/47
  In49/1 -> Mux2/48
  In50/1 -> Mux2/49
  In51/1 -> Mux2/50
  In52/1 -> Mux2/51
  In53/1 -> Mux2/52
  In54/1 -> Mux2/53
  In55/1 -> Mux2/54
  In56/1 -> Mux2/55
  In57/1 -> Mux2/56
  In58/1 -> Mux2/57
  In59/1 -> Mux2/58
  In60/1 -> Mux2/59
  In61/1 -> Mux2/60
  In62/1 -> Mux2/61
  In63/1 -> Mux2/62
  In64/1 -> Mux2/63
  In65/1 -> Mux2/64
  In66/1 -> Mux2/65
  In67/1 -> Mux2/66
  In68/1 -> Mux2/67
  In69/1 -> Mux2/68
  In70/1 -> Mux2/69
  In71/1 -> Mux2/70
  In72/1 -> Mux2/71
  In73/1 -> Mux2/72
  In74/1 -> Mux2/73
  In75/1 -> Mux2/74
  In76/1 -> Mux2/75
  In77/1 -> Mux2/76
  In78/1 -> Mux2/77
  In79/1 -> Mux2/78
  In80/1 -> Mux2/79
  In81/1 -> Mux2/80
  In82/1 -> Mux2/81
  In83/1 -> Mux2/82
  In84/1 -> Mux2/83
  In85/1 -> Mux2/84
  In86/1 -> Mux2/85
  In87/1 -> Mux2/86
  In88/1 -> Mux2/87
  In89/1 -> Mux2/88
  In90/1 -> Mux2/89
  In91/1 -> Mux2/90
  In92/1 -> Mux2/91
  In93/1 -> Mux2/92
  In94/1 -> Mux2/93
  In95/1 -> Mux2/94
  In96/1 -> Mux2/95
  In97/1 -> Mux2/96
  Mux2/1 -> Reshape2/1
  Reshape2/1 -> Cast2/1
  Cast2/1 -> Sync2/1
  Sync2/1 -> Out2/1
  In98/1 -> Cast3/1
  Cast3/1 -> Sync3/1
  Sync3/1 -> Out3/1
  In99/1 -> Cast4/1
  Cast4/1 -> Sync4/1
  Sync4/1 -> Out4/1
  In100/1 -> Cast5/1
  Cast5/1 -> Sync5/1
  Sync5/1 -> Out5/1
  In101/1 -> Cast6/1
  Cast6/1 -> Sync6/1
  Sync6/1 -> Out6/1
  In102/1 -> Cast7/1
  Cast7/1 -> Sync7/1
  Sync7/1 -> Out7/1

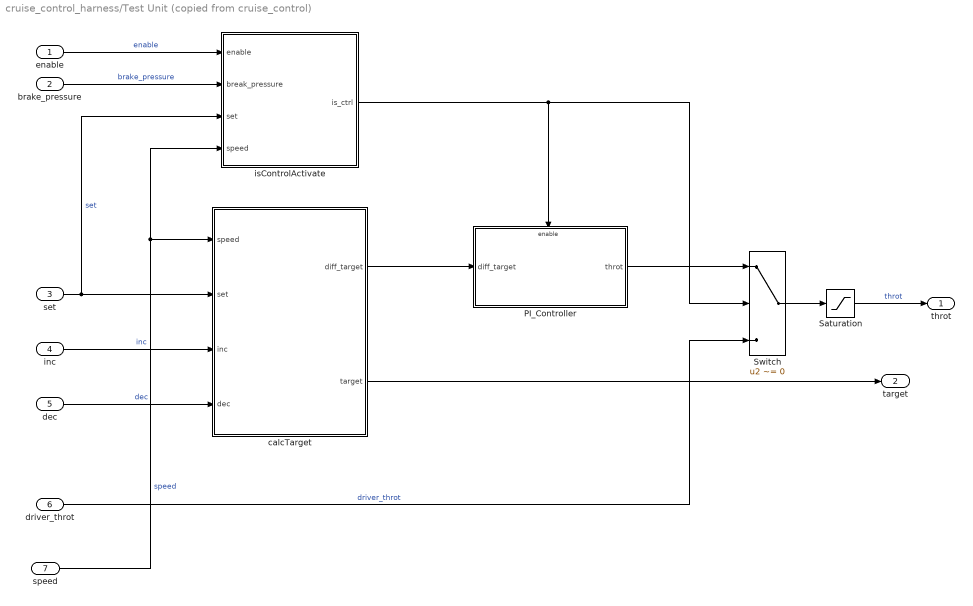
== system cruise_control_harness/Test Unit (copied from cruise_control) ==
  enable : Inport  PortDimensions=1  Interpolate=off
  brake_pressure : Inport  Port=2  PortDimensions=96  Interpolate=off
  set : Inport  Port=3  PortDimensions=1  Interpolate=off
  inc : Inport  Port=4  PortDimensions=1  Interpolate=off
  dec : Inport  Port=5  PortDimensions=1  Interpolate=off
  driver_throt : Inport  Port=6  PortDimensions=1  Interpolate=off
  speed : Inport  Port=7  PortDimensions=1  Interpolate=off
  PI_Controller : Subsystem  RequirementInfo={'other' 'cruisecontrol_spec.xls' '@Simulink_requirement_item_13' 'true' 'ƒXƒ?ƒbƒgƒ‹ŒvŽZ' '' ; 'other' 'cruisecontrol_spec.xls' '@Simulink_requirement_item_14' 'true' 'ƒXƒ?ƒbƒgƒ‹’l‚Í?API?§Œä‚É‚æ‚èŒvŽZ‚³‚ê‚é?B' '' } %GIDa_af7035a7_6314_4a61_9cdd_2b9111dd26ab
  Saturation : Saturate  RequirementInfo={'other' 'cruisecontrol_spec.xls' '@Simulink_requirement_item_15' 'true' '?o—ÍƒXƒ?ƒbƒgƒ‹’l‚Í?Å‘åƒXƒ?ƒbƒgƒ‹’lˆÈ‰º?A?Å?¬ƒXƒ?ƒbƒgƒ‹’lˆÈ?ã‚Å‚ ‚é?B' '' } %GIDa_6ec515fa_c206_4f71_9c19_d2a36a2d2cb5  UpperLimit=throt_max  LowerLimit=throt_min  OutDataTypeStr=Inherit: Inherit via back propagation
      settings: AttributesFormatString=<UpperLimit = %<UpperLimit>>\n<LowerLimit = %<LowerLimit>>
  Switch : Switch  RequirementInfo={'other' 'cruisecontrol_spec.xls' '@Simulink_requirement_item_16' 'true' '?§Œä‹–‰Â‚ªOFF‚Ì?Û‚É‚Í?Aƒhƒ‰ƒCƒo?[ƒXƒ?ƒbƒgƒ‹’l‚ªƒXƒ?ƒbƒgƒ‹’l‚Æ‚µ‚Ä?o—Í‚³‚ê‚é?B' '' } %GIDa_660ed5e2_c41f_4617_a3b9_1d6ca32493e3  Criteria=u2 ~= 0  OutDataTypeStr=Inherit: Inherit via back propagation
      settings: AttributesFormatString=<Criteria=%<Criteria>>
  calcTarget : Subsystem  RequirementInfo={'other' 'cruisecontrol_spec.xls' '@Simulink_requirement_item_4' 'true' '–Ú•WŽÔ‘¬?Ý’è' '' } %GIDa_196ed6f4_2a7d_4dba_b1ae_e2622d3b265e
  isControlActivate : Subsystem  RequirementInfo={'other' 'cruisecontrol_spec.xls' '@Simulink_requirement_item_1' 'true' 'ƒNƒ‹?[ƒYƒRƒ“ƒgƒ??[ƒ‹—LŒø‰»”»’f' '' ; 'other' 'cruisecontrol_spec.xls' '@Simulink_requirement_item_2' 'true' '?§Œä‹–‰Â‚ÍŽŸ‚Ì?ðŒ?‚ª‘S‚Ä–ž‚½‚³‚ê‚é?ê?‡‚ÉON‚Æ‚È‚é?B ?E—LŒøƒXƒCƒbƒ`‚ªON ?EƒuƒŒ?[ƒL‚ªOFF ?EƒZƒbƒgƒXƒCƒbƒ`‚ªON‚à‚µ‚­‚Í?§Œä‹–‰Â‚Ì‘O‰ñ’l‚ªON ?EŽÔ‘¬‚ª–Ú•W?Å‘åˆÈ‰º‚©‚Â?Å?¬‘¬“xˆÈ?ã' '' ; 'other' 'testsenario.xls' '@Simulink_requirement_item_1' 'true' '0' '' ; 'other' 'cruisecontrol_spec.xls' '@Simulink_requirement_item_19' 'true' 'ƒhƒ‰ƒCƒo?[ƒXƒ?ƒbƒgƒ‹’l‚Í?Å‘åƒXƒ?ƒbƒgƒ‹’lˆÈ‰º?A?Å?¬ƒXƒ?ƒbƒgƒ‹’lˆÈ?ã‚Å‚ ‚é' '' } %GIDa_e4926d79_ba1c_4fa8_ac4b_11e64dfebea6
  throt : Outport  PortDimensions=[1 1]
  target : Outport  Port=2  PortDimensions=[1 1]
  wires:
  Saturation/1 -> throt/1  "throt"
  PI_Controller/1(throt) -> Switch/1
  enable/1 -> isControlActivate/1(enable)  "enable"
  brake_pressure/1 -> isControlActivate/2(break_pressure)  "brake_pressure"
  driver_throt/1 -> Switch/3  "driver_throt"
  Switch/1 -> Saturation/1
  set/1 -> calcTarget/2(set), isControlActivate/3(set)  "set"
  inc/1 -> calcTarget/3(inc)  "inc"
  speed/1 -> calcTarget/1(speed), isControlActivate/4(speed)  "speed"
  dec/1 -> calcTarget/4(dec)  "dec"
  calcTarget/1(diff_target) -> PI_Controller/1(diff_target)
  calcTarget/2(target) -> target/1
  isControlActivate/1(is_ctrl) -> PI_Controller/Enable, Switch/2

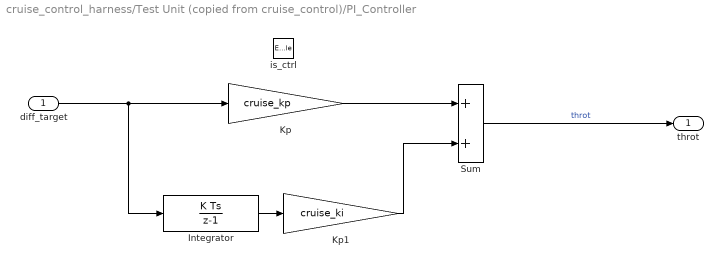
== system cruise_control_harness/Test Unit (copied from cruise_control)/PI_Controller ==
  diff_target : Inport
  is_ctrl : EnablePort  StatesWhenEnabling=reset
  Integrator : DiscreteIntegrator  RequirementInfo={'other' 'cruisecontrol_spec.xls' '@Simulink_requirement_item_18' 'true' 'ƒXƒ?ƒbƒgƒ‹’l‚Í?API?§Œä‚É‚æ‚èŒvŽZ‚³‚ê‚é?B' '' } %GIDa_c822105f_0976_492a_b1be_1f2769704f2f  gainval=1  InitialConditionMode=State only (most efficient)  SampleTime=-1  UpperSaturationLimit=5  LowerSaturationLimit=-5  ICPrevOutput=DiscIntNeverNeededParam  ICPrevScaledInput=DiscIntNeverNeededParam
      settings: AttributesFormatString=<Gain = %<gainval>>\n<%<InitialConditionMode>>\n<SampleTime = %<SampleTime>>
  Kp : Gain  RequirementInfo={'other' 'cruisecontrol_spec.xls' '@Simulink_requirement_item_18' 'true' 'ƒXƒ?ƒbƒgƒ‹’l‚Í?API?§Œä‚É‚æ‚èŒvŽZ‚³‚ê‚é?B' '' } %GIDa_0eb1e81e_39d0_414b_a305_73660988512d  Gain=cruise_kp  ParamDataTypeStr=Inherit: Inherit from 'Gain'  OutDataTypeStr=Inherit: Inherit via back propagation
  Kp1 : Gain  RequirementInfo={'other' 'cruisecontrol_spec.xls' '@Simulink_requirement_item_18' 'true' 'ƒXƒ?ƒbƒgƒ‹’l‚Í?API?§Œä‚É‚æ‚èŒvŽZ‚³‚ê‚é?B' '' } %GIDa_ed4d8c4f_5087_4321_8858_d650be1cb3fc  Gain=cruise_ki  ParamDataTypeStr=Inherit: Inherit from 'Gain'  OutDataTypeStr=Inherit: Inherit via back propagation
  Sum : Sum  RequirementInfo={'other' 'cruisecontrol_spec.xls' '@Simulink_requirement_item_18' 'true' 'ƒXƒ?ƒbƒgƒ‹’l‚Í?API?§Œä‚É‚æ‚èŒvŽZ‚³‚ê‚é?B' '' } %GIDa_04d35363_40a3_4197_b88c_74e036c86c36  OutDataTypeStr=Inherit: Inherit via back propagation
  throt : Outport  InitialOutput=0
  wires:
  Sum/1 -> throt/1  "throt"
  diff_target/1 -> Integrator/1, Kp/1
  Integrator/1 -> Kp1/1
  Kp/1 -> Sum/1
  Kp1/1 -> Sum/2

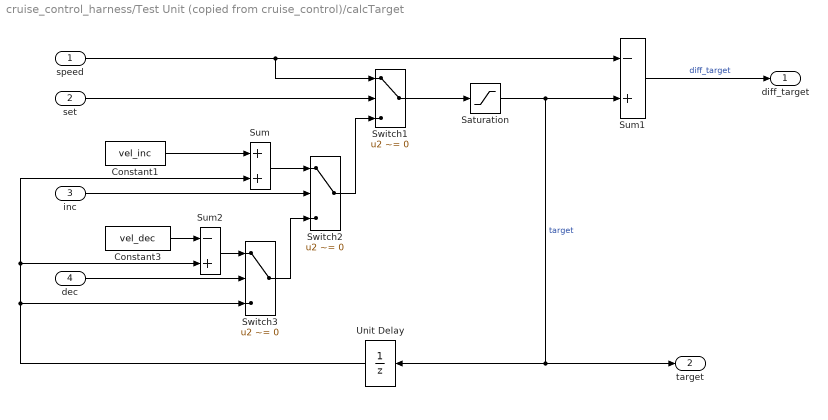
== system cruise_control_harness/Test Unit (copied from cruise_control)/calcTarget ==
  speed : Inport
  set : Inport  Port=2
  inc : Inport  Port=3
  dec : Inport  Port=4
  Constant1 : Constant  RequirementInfo={'other' 'cruisecontrol_spec.xls' '@Simulink_requirement_item_9' 'true' '‰Á‘¬ƒXƒCƒbƒ`‚ªON‚Ì?ê?‡‚É‚Í–Ú•WŽÔ‘¬‚Í‘O‰ñ’l‚É‘Î‚µ‚Ä?u‰Á‘¬’l?v‚¾‚¯‘?‰Á‚·‚é?B [?ðŒ?] ?E–Ú•WŽÔ‘¬‚Í?Å‘å‚æ‚è?¬‚©‚Â?Å?¬‚æ‚è‘å ?EƒZƒbƒgƒXƒCƒbƒ`‚ÍOFF' '' } %GIDa_ae59f12b_6370_4206_88af_856f96fce7a4  Value=vel_inc  OutDataTypeStr=Inherit: Inherit via back propagation
  Constant3 : Constant  RequirementInfo={'other' 'cruisecontrol_spec.xls' '@Simulink_requirement_item_8' 'true' 'Œ¸‘¬ƒXƒCƒbƒ`‚ªON‚Ì?ê?‡‚É‚Í–Ú•WŽÔ‘¬‚Í‘O‰ñ’l‚É‘Î‚µ‚Ä?uŒ¸‘¬’l?v‚¾‚¯Œ¸?­‚·‚é?B [?ðŒ?] ?E–Ú•WŽÔ‘¬‚Í?Å‘å‚æ‚è?¬‚©‚Â?Å?¬‚æ‚è‘å ?EƒZƒbƒgƒXƒCƒbƒ`‚ÍOFF' '' } %GIDa_a8460759_b2a2_488e_971a_4b0f1ea86130  Value=vel_dec  OutDataTypeStr=Inherit: Inherit via back propagation
  Saturation : Saturate  UpperLimit=target_max  LowerLimit=target_min
      settings: AttributesFormatString=<UpperLimit = %<UpperLimit>>\n<LowerLimit = %<LowerLimit>>
  Sum : Sum  RequirementInfo={'other' 'cruisecontrol_spec.xls' '@Simulink_requirement_item_7' 'true' '‰Á‘¬ƒXƒCƒbƒ`‚ªON‚Ì?ê?‡‚É‚Í–Ú•WŽÔ‘¬‚Í‘O‰ñ’l‚É‘Î‚µ‚Ä?u‰Á‘¬’l?v‚¾‚¯‘?‰Á‚·‚é?B [?ðŒ?] ?E–Ú•WŽÔ‘¬‚Í?Å‘å‚æ‚è?¬‚©‚Â?Å?¬‚æ‚è‘å ?EƒZƒbƒgƒXƒCƒbƒ`‚ÍOFF' '' } %GIDa_792aa8c7_f01b_4554_8eff_35efdeb3dcf2
  Sum1 : Sum  RequirementInfo={'other' 'cruisecontrol_spec.xls' '@Simulink_requirement_item_12' 'true' '–Ú•WŽÔ‘¬?·‚Í?A–Ú•WŽÔ‘¬ - ŽÔ‘¬‚Å‚ ‚é?B [‘O’ñ?ðŒ?] ?E–Ú•WŽÔ‘¬‚Í?Å‘å‚æ‚è?¬‚©‚Â?Å?¬‚æ‚è‘å' '' } %GIDa_1fe80729_51e2_4e69_a35d_769962d4f0d7  Inputs=-+  OutDataTypeStr=Inherit: Same as first input
  Sum2 : Sum  RequirementInfo={'other' 'cruisecontrol_spec.xls' '@Simulink_requirement_item_8' 'true' 'Œ¸‘¬ƒXƒCƒbƒ`‚ªON‚Ì?ê?‡‚É‚Í–Ú•WŽÔ‘¬‚Í‘O‰ñ’l‚É‘Î‚µ‚Ä?uŒ¸‘¬’l?v‚¾‚¯Œ¸?­‚·‚é?B [?ðŒ?] ?E–Ú•WŽÔ‘¬‚Í?Å‘å‚æ‚è?¬‚©‚Â?Å?¬‚æ‚è‘å ?EƒZƒbƒgƒXƒCƒbƒ`‚ÍOFF' '' } %GIDa_cee8f67d_6b1d_4448_bf19_0ab27ea0d5ea  Inputs=-+
  Switch1 : Switch  RequirementInfo={'other' 'cruisecontrol_spec.xls' '@Simulink_requirement_item_5' 'true' 'ƒZƒbƒgƒXƒCƒbƒ`‚ªON‚Ì?ê?‡‚É‚Í–Ú•WŽÔ‘¬‚ÍŒ»?Ý‚ÌŽÔ‘¬‚Æ‚È‚é [?ðŒ?] ?E–Ú•WŽÔ‘¬‚Í?Å‘å‚æ‚è?¬‚©‚Â?Å?¬‚æ‚è‘å' '' } %GIDa_86b3bc23_62e6_460b_be2f_4e3ce5376ea3  Criteria=u2 ~= 0
      settings: AttributesFormatString=<Criteria=%<Criteria>>
  Switch2 : Switch  RequirementInfo={'other' 'cruisecontrol_spec.xls' '@Simulink_requirement_item_6' 'true' 'ƒZƒbƒgƒXƒCƒbƒ`‚Í‰Á‘¬ƒXƒCƒbƒ`‚¨‚æ‚ÑŒ¸‘¬ƒXƒCƒbƒ`‚æ‚è—D?æ‚³‚ê‚é' '' ; 'other' 'cruisecontrol_spec.xls' '@Simulink_requirement_item_7' 'true' '‰Á‘¬ƒXƒCƒbƒ`‚ªON‚Ì?ê?‡‚É‚Í–Ú•WŽÔ‘¬‚Í‘O‰ñ’l‚É‘Î‚µ‚Ä?u‰Á‘¬’l?v‚¾‚¯‘?‰Á‚·‚é?B [?ðŒ?] ?E–Ú•WŽÔ‘¬‚Í?Å‘å‚æ‚è?¬‚©‚Â?Å?¬‚æ‚è‘å ?EƒZƒbƒgƒXƒCƒbƒ`‚ÍOFF' '' ; 'other' 'cruisecontrol_spec.xls' '@Simulink_requirement_item_10' 'true' '‰Á‘¬ƒXƒCƒbƒ`‚ÍŒ¸‘¬ƒXƒCƒbƒ`‚æ‚è—D?æ‚³‚ê‚é' '' } %GIDa_397a6a43_5677_411a_9718_39bb05ea81f8  Criteria=u2 ~= 0
      settings: AttributesFormatString=<Criteria=%<Criteria>>
  Switch3 : Switch  RequirementInfo={'other' 'cruisecontrol_spec.xls' '@Simulink_requirement_item_6' 'true' 'ƒZƒbƒgƒXƒCƒbƒ`‚Í‰Á‘¬ƒXƒCƒbƒ`‚¨‚æ‚ÑŒ¸‘¬ƒXƒCƒbƒ`‚æ‚è—D?æ‚³‚ê‚é' '' ; 'other' 'cruisecontrol_spec.xls' '@Simulink_requirement_item_8' 'true' 'Œ¸‘¬ƒXƒCƒbƒ`‚ªON‚Ì?ê?‡‚É‚Í–Ú•WŽÔ‘¬‚Í‘O‰ñ’l‚É‘Î‚µ‚Ä?uŒ¸‘¬’l?v‚¾‚¯Œ¸?­‚·‚é?B [?ðŒ?] ?E–Ú•WŽÔ‘¬‚Í?Å‘å‚æ‚è?¬‚©‚Â?Å?¬‚æ‚è‘å ?EƒZƒbƒgƒXƒCƒbƒ`‚ÍOFF' '' ; 'other' 'cruisecontrol_spec.xls' '@Simulink_requirement_item_10' 'true' '‰Á‘¬ƒXƒCƒbƒ`‚ÍŒ¸‘¬ƒXƒCƒbƒ`‚æ‚è—D?æ‚³‚ê‚é' '' ; 'other' 'cruisecontrol_spec.xls' '@Simulink_requirement_item_11' 'true' '‰Á‘¬ƒXƒCƒbƒ`‚¨‚æ‚ÑŒ¸‘¬ƒXƒCƒbƒ`‚ª‹¤‚É–³Œø‚Ì?ê?‡?A–Ú•WŽÔ‘¬‚Í‘O‰ñ’l‚ð—p‚¢‚é [‘O’ñ?ðŒ?] ?EƒZƒbƒgƒXƒCƒbƒ`‚ÍOFF ?E–Ú•WŽÔ‘¬‚Í?Å‘å‚æ‚è?¬‚©‚Â?Å?¬‚æ‚è‘å' '' } %GIDa_68a68a23_6ac1_4dfc_b6e0_898e041a5178  Criteria=u2 ~= 0
      settings: AttributesFormatString=<Criteria=%<Criteria>>
  Unit Delay : UnitDelay  SampleTime=-1
  diff_target : Outport
  target : Outport  Port=2
  wires:
  Sum1/1 -> diff_target/1  "diff_target"
  Switch1/1 -> Saturation/1
  Unit Delay/1 -> Sum/2, Sum2/2, Switch3/3
  Switch3/1 -> Switch2/3
  Switch2/1 -> Switch1/3
  Sum2/1 -> Switch3/1
  Constant3/1 -> Sum2/1
  dec/1 -> Switch3/2
  Sum/1 -> Switch2/1
  Constant1/1 -> Sum/1
  inc/1 -> Switch2/2
  speed/1 -> Sum1/1, Switch1/1
  set/1 -> Switch1/2
  Saturation/1 -> Unit Delay/1, target/1, Sum1/2  "target"

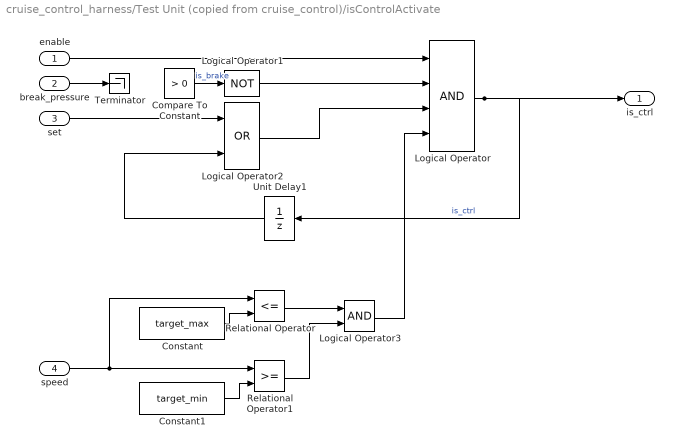
== system cruise_control_harness/Test Unit (copied from cruise_control)/isControlActivate ==
  enable : Inport
  break_pressure : Inport  Port=2
  set : Inport  Port=3
  speed : Inport  Port=4
  Compare To Constant : simulink/Logic and Bit Operations/Compare To Constant  RequirementInfo={'other' 'cruisecontrol_spec.xls' '@Simulink_requirement_item_17' 'true' '?§Œä‹–‰Â‚ÍŽŸ‚Ì?ðŒ?‚ª‘S‚Ä–ž‚½‚³‚ê‚é?ê?‡‚ÉON‚Æ‚È‚é?B ?E—LŒøƒXƒCƒbƒ`‚ªON ?EƒuƒŒ?[ƒL‚ªOFF ?EƒZƒbƒgƒXƒCƒbƒ`‚ªON‚à‚µ‚­‚Í?§Œä‹–‰Â‚Ì‘O‰ñ’l‚ªON ?EŽÔ‘¬‚ª–Ú•W?Å‘åˆÈ‰º‚©‚Â?Å?¬‘¬“xˆÈ?ã' '' } %GIDa_19f09b28_2ee5_4051_af8a_4fb6ece4e2eb  relop=>  const=0  OutDataTypeStr=uint8
  Constant : Constant  RequirementInfo={'other' 'cruisecontrol_spec.xls' '@Simulink_requirement_item_17' 'true' '?§Œä‹–‰Â‚ÍŽŸ‚Ì?ðŒ?‚ª‘S‚Ä–ž‚½‚³‚ê‚é?ê?‡‚ÉON‚Æ‚È‚é?B ?E—LŒøƒXƒCƒbƒ`‚ªON ?EƒuƒŒ?[ƒL‚ªOFF ?EƒZƒbƒgƒXƒCƒbƒ`‚ªON‚à‚µ‚­‚Í?§Œä‹–‰Â‚Ì‘O‰ñ’l‚ªON ?EŽÔ‘¬‚ª–Ú•W?Å‘åˆÈ‰º‚©‚Â?Å?¬‘¬“xˆÈ?ã' '' } %GIDa_f55cf62f_5fc4_4dcd_845b_cc89100af1fb  Value=target_max
  Constant1 : Constant  RequirementInfo={'other' 'cruisecontrol_spec.xls' '@Simulink_requirement_item_17' 'true' '?§Œä‹–‰Â‚ÍŽŸ‚Ì?ðŒ?‚ª‘S‚Ä–ž‚½‚³‚ê‚é?ê?‡‚ÉON‚Æ‚È‚é?B ?E—LŒøƒXƒCƒbƒ`‚ªON ?EƒuƒŒ?[ƒL‚ªOFF ?EƒZƒbƒgƒXƒCƒbƒ`‚ªON‚à‚µ‚­‚Í?§Œä‹–‰Â‚Ì‘O‰ñ’l‚ªON ?EŽÔ‘¬‚ª–Ú•W?Å‘åˆÈ‰º‚©‚Â?Å?¬‘¬“xˆÈ?ã' '' } %GIDa_88bdc187_6186_4b2e_b486_b87bd0da6e54  Value=target_min
  Logical Operator : Logic  RequirementInfo={'other' 'cruisecontrol_spec.xls' '@Simulink_requirement_item_17' 'true' '?§Œä‹–‰Â‚ÍŽŸ‚Ì?ðŒ?‚ª‘S‚Ä–ž‚½‚³‚ê‚é?ê?‡‚ÉON‚Æ‚È‚é?B ?E—LŒøƒXƒCƒbƒ`‚ªON ?EƒuƒŒ?[ƒL‚ªOFF ?EƒZƒbƒgƒXƒCƒbƒ`‚ªON‚à‚µ‚­‚Í?§Œä‹–‰Â‚Ì‘O‰ñ’l‚ªON ?EŽÔ‘¬‚ª–Ú•W?Å‘åˆÈ‰º‚©‚Â?Å?¬‘¬“xˆÈ?ã' '' } %GIDa_6924fecc_2500_4d6b_afec_01e6803cf191  Inputs=4  AllPortsSameDT=off  OutDataTypeStr=boolean
  Logical Operator1 : Logic  RequirementInfo={'other' 'cruisecontrol_spec.xls' '@Simulink_requirement_item_17' 'true' '?§Œä‹–‰Â‚ÍŽŸ‚Ì?ðŒ?‚ª‘S‚Ä–ž‚½‚³‚ê‚é?ê?‡‚ÉON‚Æ‚È‚é?B ?E—LŒøƒXƒCƒbƒ`‚ªON ?EƒuƒŒ?[ƒL‚ªOFF ?EƒZƒbƒgƒXƒCƒbƒ`‚ªON‚à‚µ‚­‚Í?§Œä‹–‰Â‚Ì‘O‰ñ’l‚ªON ?EŽÔ‘¬‚ª–Ú•W?Å‘åˆÈ‰º‚©‚Â?Å?¬‘¬“xˆÈ?ã' '' } %GIDa_37138771_8436_4632_bb6c_d34928288879  Operator=NOT  AllPortsSameDT=off  OutDataTypeStr=boolean
  Logical Operator2 : Logic  RequirementInfo={'other' 'cruisecontrol_spec.xls' '@Simulink_requirement_item_17' 'true' '?§Œä‹–‰Â‚ÍŽŸ‚Ì?ðŒ?‚ª‘S‚Ä–ž‚½‚³‚ê‚é?ê?‡‚ÉON‚Æ‚È‚é?B ?E—LŒøƒXƒCƒbƒ`‚ªON ?EƒuƒŒ?[ƒL‚ªOFF ?EƒZƒbƒgƒXƒCƒbƒ`‚ªON‚à‚µ‚­‚Í?§Œä‹–‰Â‚Ì‘O‰ñ’l‚ªON ?EŽÔ‘¬‚ª–Ú•W?Å‘åˆÈ‰º‚©‚Â?Å?¬‘¬“xˆÈ?ã' '' } %GIDa_78a97924_986a_4892_aca5_0f2e6241b780  Operator=OR  AllPortsSameDT=off  OutDataTypeStr=boolean
  Logical Operator3 : Logic  RequirementInfo={'other' 'cruisecontrol_spec.xls' '@Simulink_requirement_item_17' 'true' '?§Œä‹–‰Â‚ÍŽŸ‚Ì?ðŒ?‚ª‘S‚Ä–ž‚½‚³‚ê‚é?ê?‡‚ÉON‚Æ‚È‚é?B ?E—LŒøƒXƒCƒbƒ`‚ªON ?EƒuƒŒ?[ƒL‚ªOFF ?EƒZƒbƒgƒXƒCƒbƒ`‚ªON‚à‚µ‚­‚Í?§Œä‹–‰Â‚Ì‘O‰ñ’l‚ªON ?EŽÔ‘¬‚ª–Ú•W?Å‘åˆÈ‰º‚©‚Â?Å?¬‘¬“xˆÈ?ã' '' } %GIDa_55c027f9_c8c8_4e05_a082_e1b4fc2bab81  AllPortsSameDT=off  OutDataTypeStr=boolean
  Relational Operator : RelationalOperator  RequirementInfo={'other' 'cruisecontrol_spec.xls' '@Simulink_requirement_item_17' 'true' '?§Œä‹–‰Â‚ÍŽŸ‚Ì?ðŒ?‚ª‘S‚Ä–ž‚½‚³‚ê‚é?ê?‡‚ÉON‚Æ‚È‚é?B ?E—LŒøƒXƒCƒbƒ`‚ªON ?EƒuƒŒ?[ƒL‚ªOFF ?EƒZƒbƒgƒXƒCƒbƒ`‚ªON‚à‚µ‚­‚Í?§Œä‹–‰Â‚Ì‘O‰ñ’l‚ªON ?EŽÔ‘¬‚ª–Ú•W?Å‘åˆÈ‰º‚©‚Â?Å?¬‘¬“xˆÈ?ã' '' } %GIDa_28848ad3_2d02_4c4e_8895_07262833c089  Operator=<=  OutDataTypeStr=boolean
  Relational Operator1 : RelationalOperator  RequirementInfo={'other' 'cruisecontrol_spec.xls' '@Simulink_requirement_item_17' 'true' '?§Œä‹–‰Â‚ÍŽŸ‚Ì?ðŒ?‚ª‘S‚Ä–ž‚½‚³‚ê‚é?ê?‡‚ÉON‚Æ‚È‚é?B ?E—LŒøƒXƒCƒbƒ`‚ªON ?EƒuƒŒ?[ƒL‚ªOFF ?EƒZƒbƒgƒXƒCƒbƒ`‚ªON‚à‚µ‚­‚Í?§Œä‹–‰Â‚Ì‘O‰ñ’l‚ªON ?EŽÔ‘¬‚ª–Ú•W?Å‘åˆÈ‰º‚©‚Â?Å?¬‘¬“xˆÈ?ã' '' } %GIDa_74fb8f9b_346c_4d62_8293_c5d1c796f058  OutDataTypeStr=boolean
  Terminator : Terminator
  Unit Delay1 : UnitDelay  RequirementInfo={'other' 'cruisecontrol_spec.xls' '@Simulink_requirement_item_3' 'true' '?‰Šú?ðŒ?‚Å‚ÍƒZƒbƒgƒXƒCƒbƒ`‚ªON‚Å‚È‚¢ŒÀ‚è?§Œä‹–‰Â‚Í–³Œø‚Å‚ ‚é' '' } %GIDa_e39c0747_4cc6_4769_b8d5_a7f6526c8e0b  SampleTime=-1
  is_ctrl : Outport
  wires:
  break_pressure/1 -> Terminator/1
  Logical Operator/1 -> Unit Delay1/1, is_ctrl/1  "is_ctrl"
  Unit Delay1/1 -> Logical Operator2/2
  Logical Operator2/1 -> Logical Operator/3
  Logical Operator1/1 -> Logical Operator/2
  set/1 -> Logical Operator2/1
  enable/1 -> Logical Operator/1
  Constant1/1 -> Relational Operator1/2
  speed/1 -> Relational Operator1/1, Relational Operator/1
  Relational Operator/1 -> Logical Operator3/1
  Relational Operator1/1 -> Logical Operator3/2
  Logical Operator3/1 -> Logical Operator/4
  Constant/1 -> Relational Operator/2
  Compare To Constant/1 -> Logical Operator1/1  "is_brake"
